simulink model "Mo_hinh_khoi_dong_3_cap_toc_do"  (R2019a)
settings: Solver=VariableStepAuto  StartTime=0.0  StopTime=10.0  RelTol=1e-3
libraries: powerlib x17, simulink x1
settings Model: Creator=trung  LastModifiedBy=Admin
settings DataIOCC: ReturnWorkspaceOutputs=off
settings DebuggingCC: PregeneratedLibrarySubsystemCodeDiagnostic=none  ArithmeticOperatorsInVariantConditions=warning
settings SFSimCC: SimUseLocalCustomCode=off
settings RTWCC: RTWUseLocalCustomCode=off

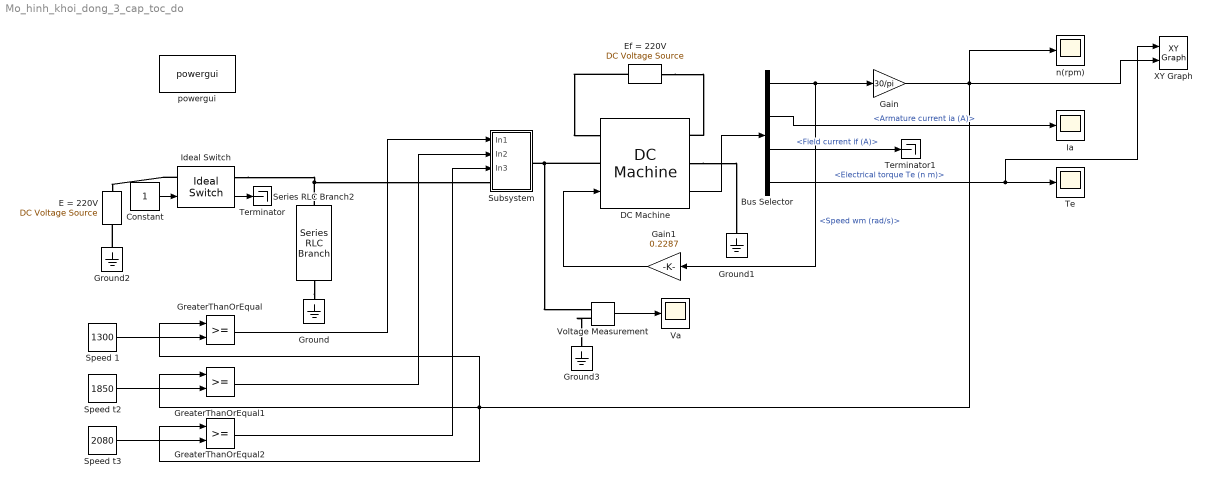
== system Mo_hinh_khoi_dong_3_cap_toc_do ==
  Bus Selector : BusSelector  OutputSignals=Speed wm (rad/s),Armature current ia (A),Field current if (A),Electrical torque Te (n m)
  Constant : Constant
  DC Machine : powerlib/Machines/DC Machine  PresetModel=No  MechanicalLoad=Torque TL  FieldType=Wound  ShowDetailedParameters=on  MeasurementBus=off  RLa=[0.2305 0.023]  RLf=[298 59.6]  Laf=1.247  MachineConstant=Torque constant (N.m/A)  Ke=1.8  Kt=1.8  J=0.28  Bm=1.58e-4  Tf=1.75  w0=1  Ifinit=1  TsPowergui=0  TsBlock=-1
      settings: SourceProductName=Simscape Electrical
  E = 220V : powerlib/Electrical Sources/DC Voltage Source  Amplitude=220  Measurements=None
      settings: SourceProductName=Simscape Electrical
  Ef = 220V : powerlib/Electrical Sources/DC Voltage Source  Amplitude=220  Measurements=None
      settings: SourceProductName=Simscape Electrical
  Gain : Gain  Gain=30/pi
  Gain1 : Gain  Gain=0.2287
  GreaterThanOrEqual : RelationalOperator  OutDataTypeStr=boolean  RndMeth=Simplest
  GreaterThanOrEqual1 : RelationalOperator  OutDataTypeStr=boolean  RndMeth=Simplest
  GreaterThanOrEqual2 : RelationalOperator  OutDataTypeStr=boolean  RndMeth=Simplest
  Ground{,1..3} (4 alike) : powerlib/Elements/Ground  LConnTagsString=a
      settings: SourceProductName=Simscape Electrical
  Ia : Scope
  Ideal Switch : powerlib/Power Electronics/Ideal Switch  Ron=0.01  Lon=0  IC=0  Rs=inf  Cs=0  Measurements=on
      settings: SourceProductName=Simscape Electrical
  Series RLC Branch2 : powerlib/Elements/Series RLC Branch  LConnTagsString=__new0  RConnTagsString=__new0  BranchType=R  Resistance=10000  Inductance=1e-3  SetiL0=off  InitialCurrent=0  Capacitance=1e-6  Setx0=off  InitialVoltage=0  Measurements=None
      settings: SourceProductName=Simscape Electrical
  "Speed 1 " : Constant  Value=1300
  Speed t2 : Constant  Value=1850
  Speed t3 : Constant  Value=2080
  Subsystem : Subsystem
  Te : Scope
  Terminator : Terminator
  Terminator1 : Terminator
  "Va " : Scope
  Voltage Measurement : powerlib/Measurements/Voltage Measurement  PhasorSimulation=off  OutputType=Complex  PSBequivalent=0
      settings: SourceProductName=Simscape Electrical
  XY Graph : simulink/Sinks/XY Graph  xmin=0  xmax=200  ymin=-2500  ymax=2500  st=-1
  "n(rpm) " : Scope
  powergui : powerlib/powergui  Priority=1  SimulationMode=Continuous  SampleTime=50e-6  frequency=60  Iterations=50  frequencyindice=0  Pbase=100e6  ErrMax=1e-4  UnitsV=kV  UnitsW=MW  buscounter=0  FunctionMessages=off  echomessages=off  EnableUseOfTLC=off  CurrentSourceSwitches=off  DisableSnubberDevices=off  DisableRonSwitches=off  DisableVfSwitches=off  DisplayEquations=off  AutomaticDiscreteSolvers=off  SolverType=Tustin/Backward Euler (TBE)  Interpol=off  ExternalGateDelay=off  methode=off  Ts=100  x0status=blocks  SPID=on  SwTol=0  HookPort=off  NonlinearTolerance=0  nMaxIteration=15  ContinueOnMaxIteration=off  RestoreLinks=warning  ResistiveCurrentMeasurement=off  Frange=[0:2:500]  Ylog=off  Xlog=on  ShowGrid=off  save=off  variable=ZData  structure=0  ZoomFFT=off  StartTime=0.0  cycles=1  DisplayStyle=1  fundamental=60  FreqAxis=off  MaxFrequency=1000  frequencyindicesteady=1  RmsSteady=1  display=off
      settings: SourceProductName=Simscape Electrical
  wires:
  Voltage Measurement/1 -> "Va "/1
  Gain1/1 -> DC Machine/1
  Bus Selector/2 -> Ia/1  "<Armature current ia (A)>"
  Bus Selector/4 -> XY Graph/1, Te/1  "<Electrical torque Te (n m)>"
  DC Machine/1 -> Bus Selector/1
  Ideal Switch/1 -> Terminator/1
  Bus Selector/1 -> Gain1/1, Gain/1  "<Speed wm (rad/s)>"
  Bus Selector/3 -> Terminator1/1  "<Field current if (A)>"
  Gain/1 -> XY Graph/2, GreaterThanOrEqual2/1, GreaterThanOrEqual/1, GreaterThanOrEqual1/1, "n(rpm) "/1
  Constant/1 -> Ideal Switch/1
  "Speed 1 "/1 -> GreaterThanOrEqual/2
  Speed t2/1 -> GreaterThanOrEqual1/2
  Speed t3/1 -> GreaterThanOrEqual2/2
  GreaterThanOrEqual/1 -> Subsystem/1(In1)
  GreaterThanOrEqual1/1 -> Subsystem/2(In2)
  GreaterThanOrEqual2/1 -> Subsystem/3(In3)
  connections:
  Voltage Measurement/LConn2 -- Ground3/LConn1
  Ef = 220V/RConn1 -- DC Machine/LConn2
  Ef = 220V/LConn1 -- DC Machine/RConn2
  Ground2/LConn1 -- E = 220V/LConn1
  Ideal Switch/LConn1 -- E = 220V/RConn1
  DC Machine/RConn1 -- Ground1/LConn1
  Series RLC Branch2/LConn1 -- Ideal Switch/RConn1 -- Subsystem/LConn1
  DC Machine/LConn1 -- Voltage Measurement/LConn1 -- Subsystem/RConn1
  Series RLC Branch2/RConn1 -- Ground/LConn1

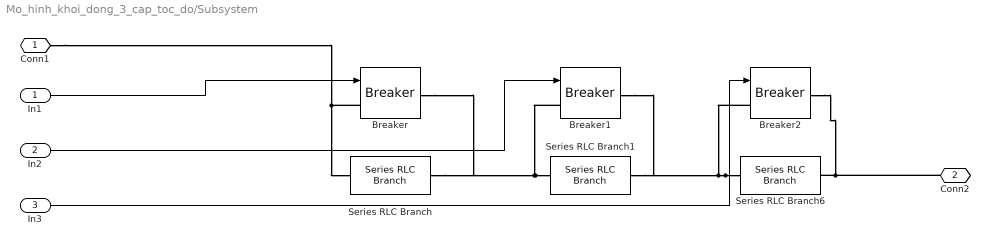
== system Mo_hinh_khoi_dong_3_cap_toc_do/Subsystem ==
  In1 : Inport
  In2 : Inport  Port=2
  In3 : Inport  Port=3
  Breaker : powerlib/Elements/Breaker  InitialState=0  SwitchingTimes="[1/60  5/60]"  External=on  BreakerResistance=0.01  SnubberResistance=1e6  SnubberCapacitance=inf  Measurements=None  MoreParameters=on  NoBreakLoop=off
      settings: SourceProductName=Simscape Electrical
  Breaker1 : powerlib/Elements/Breaker  InitialState=0  SwitchingTimes="[1/60  5/60]"  External=on  BreakerResistance=0.01  SnubberResistance=1e6  SnubberCapacitance=inf  Measurements=None  MoreParameters=on  NoBreakLoop=off
      settings: SourceProductName=Simscape Electrical
  Breaker2 : powerlib/Elements/Breaker  InitialState=0  SwitchingTimes="[1/60  5/60]"  External=on  BreakerResistance=0.01  SnubberResistance=1e6  SnubberCapacitance=inf  Measurements=None  MoreParameters=on  NoBreakLoop=off
      settings: SourceProductName=Simscape Electrical
  Series RLC Branch : powerlib/Elements/Series RLC Branch  LConnTagsString=__new0  RConnTagsString=__new0  BranchType=R  Resistance=0.366  Inductance=1e-3  SetiL0=off  InitialCurrent=0  Capacitance=1e-6  Setx0=off  InitialVoltage=0  Measurements=None
      settings: SourceProductName=Simscape Electrical
  Series RLC Branch1 : powerlib/Elements/Series RLC Branch  LConnTagsString=__new0  RConnTagsString=__new0  BranchType=R  Resistance=0.164  Inductance=1e-3  SetiL0=off  InitialCurrent=0  Capacitance=1e-6  Setx0=off  InitialVoltage=0  Measurements=None
      settings: SourceProductName=Simscape Electrical
  Series RLC Branch6 : powerlib/Elements/Series RLC Branch  LConnTagsString=__new0  RConnTagsString=__new0  BranchType=R  Resistance=0.074  Inductance=1e-3  SetiL0=off  InitialCurrent=0  Capacitance=1e-6  Setx0=off  InitialVoltage=0  Measurements=None
      settings: SourceProductName=Simscape Electrical
  Conn1 : PMIOPort  Side=Left
  Conn2 : PMIOPort  Port=2  Side=Right
  wires:
  In3/1 -> Breaker2/1
  In2/1 -> Breaker1/1
  In1/1 -> Breaker/1
  connections:
  Breaker/LConn1 -- Series RLC Branch/LConn1 -- Conn1/RConn1
  Series RLC Branch6/RConn1 -- Breaker2/RConn1 -- Conn2/RConn1
  Series RLC Branch6/LConn1 -- Breaker2/LConn1 -- Series RLC Branch1/RConn1 -- Breaker1/RConn1
  Series RLC Branch1/LConn1 -- Breaker1/LConn1 -- Series RLC Branch/RConn1 -- Breaker/RConn1
